simulink model "PIDcontrollerv2"  (R2018b)
settings: Solver=VariableStepAuto  StartTime=0.0  StopTime=20  RelTol=1e-3
libraries: simulink x1
settings Model: Creator=KaSat  LastModifiedBy=KaSat

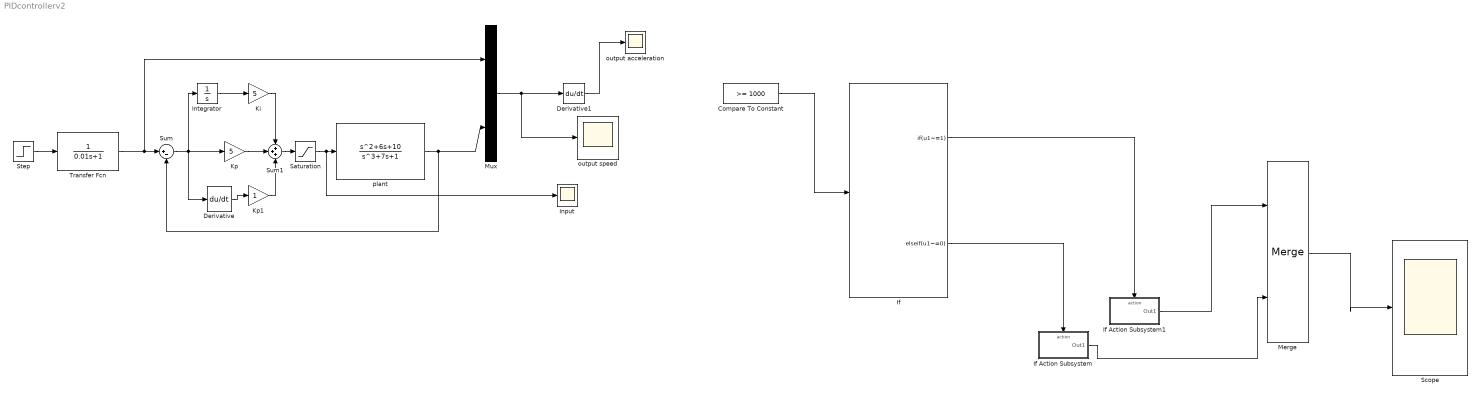
== system PIDcontrollerv2 ==
  Compare To Constant : simulink/Logic and Bit Operations/Compare To Constant  relop=>=  const=1000  OutDataTypeStr=boolean
  Derivative : Derivative
  Derivative1 : Derivative
  If : If  IfExpression=u1~=1  ElseIfExpressions=u1~=0  ShowElse=off
  If Action Subsystem : Subsystem  TreatAsAtomicUnit=on
  If Action Subsystem1 : Subsystem  TreatAsAtomicUnit=on
  Input : Scope
  Integrator : Integrator
  Ki : Gain  Gain=5
  Kp : Gain  Gain=5
  Kp1 : Gain
  Merge : Merge
  Mux : Mux  Inputs=2
  Saturation : Saturate  UpperLimit=10  LowerLimit=-10
  Scope : Scope
  "Step " : Step  SampleTime=0
  Sum : Sum  Inputs=|+-
  Sum1 : Sum  Inputs=+++
  Transfer Fcn : TransferFcn  Denominator=[0.01 1]
  output acceleration : Scope
  output speed : Scope
  plant : TransferFcn  Numerator=[1,6,10]  Denominator=[1,0,7,1]
  wires:
  plant/1 -> Mux/2, Sum/2
  Sum/1 -> Derivative/1, Integrator/1, Kp/1
  Mux/1 -> output speed/1, Derivative1/1
  Integrator/1 -> Ki/1
  Kp/1 -> Sum1/2
  Ki/1 -> Sum1/1
  Derivative/1 -> Kp1/1
  Kp1/1 -> Sum1/3
  "Step "/1 -> Transfer Fcn/1
  Transfer Fcn/1 -> Mux/1, Sum/1
  Sum1/1 -> Saturation/1
  Saturation/1 -> Input/1, plant/1
  Derivative1/1 -> output acceleration/1
  Compare To Constant/1 -> If/1
  If/2 -> If Action Subsystem/Action
  If/1 -> If Action Subsystem1/Action
  If Action Subsystem1/1(Out1) -> Merge/1
  If Action Subsystem/1(Out1) -> Merge/2
  Merge/1 -> Scope/1

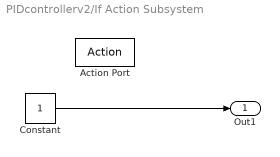
== system PIDcontrollerv2/If Action Subsystem ==
  Action Port : ActionPort  ActionType=elseif
  Constant : Constant
  Out1 : Outport
  wires:
  Constant/1 -> Out1/1

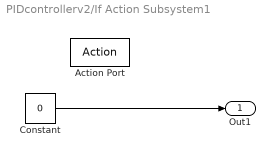
== system PIDcontrollerv2/If Action Subsystem1 ==
  Action Port : ActionPort  ActionType=then
  Constant : Constant  Value=0
  Out1 : Outport
  wires:
  Constant/1 -> Out1/1
